simulink library "INT_EGRVlv_VDPosGov"  (R2016b)
settings: Solver=VariableStepAuto  StartTime=0.0  StopTime=10.0  RelTol=1e-3
settings Model: Creator=zhoutinglin  LastModifiedBy=zhoutinglin

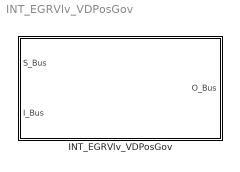
== system INT_EGRVlv_VDPosGov ==
  INT_EGRVlv_VDPosGov : Subsystem

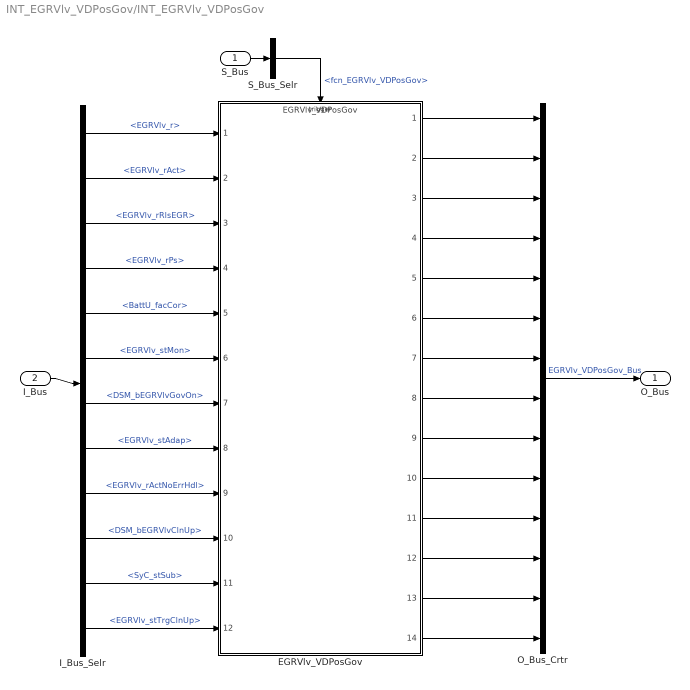
== system INT_EGRVlv_VDPosGov/INT_EGRVlv_VDPosGov ==
  S_Bus : Inport
  I_Bus : Inport  Port=2
  EGRVlv_VDPosGov : ModelReference  ModelNameDialog=EGRVlv_VDPosGov  SimulationMode=Normal  ModelReferenceVersion=1.26  TriggerPortName=function  TriggerPortTriggerType=function-call  TriggerPortStatesWhenEnabling=held
  I_Bus_Selr : BusSelector  OutputSignals=EGRVlv_r,EGRVlv_rAct,EGRVlv_rRlsEGR,EGRVlv_rPs,BattU_facCor,EGRVlv_stMon,DSM_bEGRVlvGovOn,EGRVlv_stAdap,EGRVlv_rActNoErrHdl,DSM_bEGRVlvClnUp,SyC_stSub,EGRVlv_stTrgClnUp
  O_Bus_Crtr : BusCreator  Inputs=14
  S_Bus_Selr : BusSelector  OutputSignals=fcn_EGRVlv_VDPosGov
  O_Bus : Outport
  wires:
  S_Bus_Selr/1 -> EGRVlv_VDPosGov/Trigger  "<fcn_EGRVlv_VDPosGov>"
  S_Bus/1 -> S_Bus_Selr/1
  I_Bus/1 -> I_Bus_Selr/1
  I_Bus_Selr/1 -> EGRVlv_VDPosGov/1  "<EGRVlv_r>"
  I_Bus_Selr/2 -> EGRVlv_VDPosGov/2  "<EGRVlv_rAct>"
  I_Bus_Selr/3 -> EGRVlv_VDPosGov/3  "<EGRVlv_rRlsEGR>"
  I_Bus_Selr/4 -> EGRVlv_VDPosGov/4  "<EGRVlv_rPs>"
  I_Bus_Selr/5 -> EGRVlv_VDPosGov/5  "<BattU_facCor>"
  I_Bus_Selr/6 -> EGRVlv_VDPosGov/6  "<EGRVlv_stMon>"
  I_Bus_Selr/7 -> EGRVlv_VDPosGov/7  "<DSM_bEGRVlvGovOn>"
  I_Bus_Selr/8 -> EGRVlv_VDPosGov/8  "<EGRVlv_stAdap>"
  I_Bus_Selr/9 -> EGRVlv_VDPosGov/9  "<EGRVlv_rActNoErrHdl>"
  I_Bus_Selr/10 -> EGRVlv_VDPosGov/10  "<DSM_bEGRVlvClnUp>"
  I_Bus_Selr/11 -> EGRVlv_VDPosGov/11  "<SyC_stSub>"
  I_Bus_Selr/12 -> EGRVlv_VDPosGov/12  "<EGRVlv_stTrgClnUp>"
  O_Bus_Crtr/1 -> O_Bus/1  "EGRVlv_VDPosGov_Bus"
  EGRVlv_VDPosGov/1 -> O_Bus_Crtr/1
  EGRVlv_VDPosGov/2 -> O_Bus_Crtr/2
  EGRVlv_VDPosGov/3 -> O_Bus_Crtr/3
  EGRVlv_VDPosGov/4 -> O_Bus_Crtr/4
  EGRVlv_VDPosGov/5 -> O_Bus_Crtr/5
  EGRVlv_VDPosGov/6 -> O_Bus_Crtr/6
  EGRVlv_VDPosGov/7 -> O_Bus_Crtr/7
  EGRVlv_VDPosGov/8 -> O_Bus_Crtr/8
  EGRVlv_VDPosGov/9 -> O_Bus_Crtr/9
  EGRVlv_VDPosGov/10 -> O_Bus_Crtr/10
  EGRVlv_VDPosGov/11 -> O_Bus_Crtr/11
  EGRVlv_VDPosGov/12 -> O_Bus_Crtr/12
  EGRVlv_VDPosGov/13 -> O_Bus_Crtr/13
  EGRVlv_VDPosGov/14 -> O_Bus_Crtr/14
